simulink model "Teste_Paper_Malha_Aceleracao"  (R2013b)
settings: Solver=ode45  StartTime=0.0  StopTime=10  RelTol=1e-3
values from neighbouring files (symbols this model uses):
  A = zeros(n, n)    [Lineariza.m]    (also in MatrizesDeEstado.mat = [-0.0193051557459 -0.000253889151844 -1.42063941966e-10 0 0 ; SimulacaoLinear.m = A(1:12,1:12); comparacao_paper.m = An; teste_Controlador_LateroDirecional.m = A_lat{k})
  Aad = p.a    [comparacao_paper.m]
  B = zeros(n, mm)    [Lineariza.m]    (also in MatrizesDeEstado.mat = [0 0 0 0 0 0 0 0 0 0 0 0 ... (52 elements, 13x4)]; SimulacaoLinear.m = B(1:12, 2:end); comparacao_paper.m = Bn; teste_Controlador_LateroDirecional.m = B_lat{k})
  Bad = p.b    [comparacao_paper.m]
  C = zeros(saidas, n)    [Lineariza.m]    (also in MatrizesDeEstado.mat = [0 0.00398133423863 0.00398133423863 0 16.2830679635 16.2830; SimulacaoLinear.m = eye(max(size(A))); comparacao_paper.m = Cn; teste_Controlador_LateroDirecional.m = [0 1 0 0)
  Cad = p.c    [comparacao_paper.m]
  D = zeros(saidas, mm)    [Lineariza.m]    (also in MatrizesDeEstado.mat = [0  0  0  0; 0  -0.0485273813531  0  0; 0  -0.0485273813531 ; SimulacaoLinear.m = zeros(12,3); comparacao_paper.m = Dn; teste_Controlador_LateroDirecional.m = [0 0)
  Dad = p.d    [comparacao_paper.m]
  k_i = T.Blocks.ki.Value    [comparacao_paper.m]
  k_p = T.Blocks.kp.Value    [comparacao_paper.m]
  k_q = T.Blocks.kq.Value    [comparacao_paper.m]
settings Model: Creator=Eduardo  LastModifiedBy=Eduardo

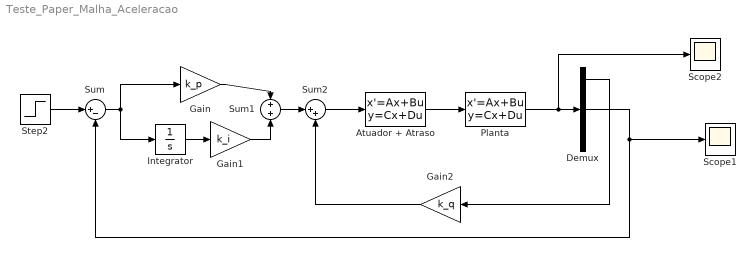
== system Teste_Paper_Malha_Aceleracao ==
  Atuador + Atraso : StateSpace  A=Aad  B=Bad  C=Cad  D=Dad  X0=0
  Demux : Demux  Outputs=3
  Gain : Gain  Gain=k_p
  Gain1 : Gain  Gain=k_i
  Gain2 : Gain  Gain=k_q
  Integrator : Integrator
  Planta : StateSpace  A=A  B=B  C=C  D=D  X0=0
  Scope1 : Scope
  Scope2 : Scope
      settings: SaveName=ScopeData2
  Step2 : Step  SampleTime=0
  Sum : Sum  Inputs=|+-
  Sum1 : Sum  Inputs=+|+
  Sum2 : Sum  Inputs=|++
  wires:
  Integrator/1 -> Gain1/1
  Gain/1 -> Sum1/1
  Gain1/1 -> Sum1/2
  Planta/1 -> Demux/1, Scope2/1
  Step2/1 -> Sum/1
  Sum/1 -> Gain/1, Integrator/1
  Demux/1 -> Gain2/1
  Demux/2 -> Scope1/1, Sum/2
  Sum1/1 -> Sum2/1
  Sum2/1 -> Atuador + Atraso/1
  Gain2/1 -> Sum2/2
  Atuador + Atraso/1 -> Planta/1
